simulink model "FF_generator"  (R2020b)
settings: Solver=FixedStepAuto  StartTime=0.0  StopTime=120  FixedStep=1e-5  RelTol=1e-3
libraries: simulink x1
settings Model: Creator=oboe  LastModifiedBy=reglab
settings DataIOCC: ReturnWorkspaceOutputs=off
settings DebuggingCC: ArithmeticOperatorsInVariantConditions=warning
settings SFSimCC: SimUseLocalCustomCode=off  CustomCodeUndefinedFunction=UseInterfaceOnly
settings RTWCC: RTWUseLocalCustomCode=off
settings CodeAppCC: StateflowObjectComments=on

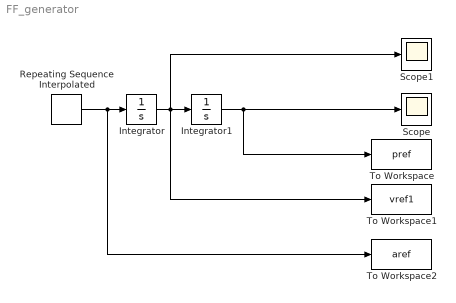
== system FF_generator ==
  Integrator : Integrator
  Integrator1 : Integrator
  Repeating Sequence Interpolated : simulink/Sources/Repeating Sequence Interpolated  OutValues=[0 0 1 1 0 0 -1 -1 0 0 -1*[0 0 1 1 0 0 -1 -1 0 0]].'  TimeValues=[0 1 1.0000001 1.5 1.50000001 4.5 4.50000001 5 5.0000001 6 6+[0.0000001 1 1.0000001 1.5 1.50000001 4.5 4.50000001 5 5.0000001 6]].'  LookUpMeth=Interpolation-Use End Values  tsamp=0.002  OutMin=[]  OutMax=[]  OutDataTypeStr=double  OutputDataTypeScalingMode=double  OutDataType=fixdt(0,8)  OutScaling=2^-10
  Scope : Scope
  Scope1 : Scope
  To Workspace : ToWorkspace  VariableName=pref  SaveFormat=Structure With Time  SampleTime=.001
  To Workspace1 : ToWorkspace  VariableName=vref1  SaveFormat=Structure With Time  SampleTime=.001
  To Workspace2 : ToWorkspace  VariableName=aref  SaveFormat=Structure With Time  SampleTime=.001
  wires:
  Integrator1/1 -> To Workspace/1, Scope/1
  Integrator/1 -> To Workspace1/1, Scope1/1, Integrator1/1
  Repeating Sequence Interpolated/1 -> To Workspace2/1, Integrator/1
